simulink model "single_track"  (R2022b)
settings: Solver=VariableStepAuto  StartTime=0.0  StopTime=30  RelTol=1e-5
libraries: autolibshared x1
settings Model: Creator=ashkan  LastModifiedBy=ashkan

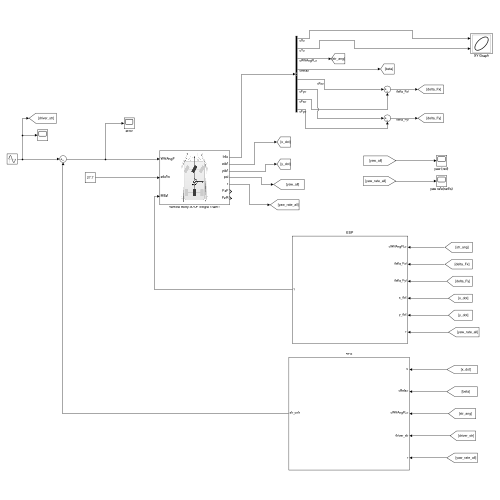
[thumbnail: Simulink's stored preview of the top-level diagram]
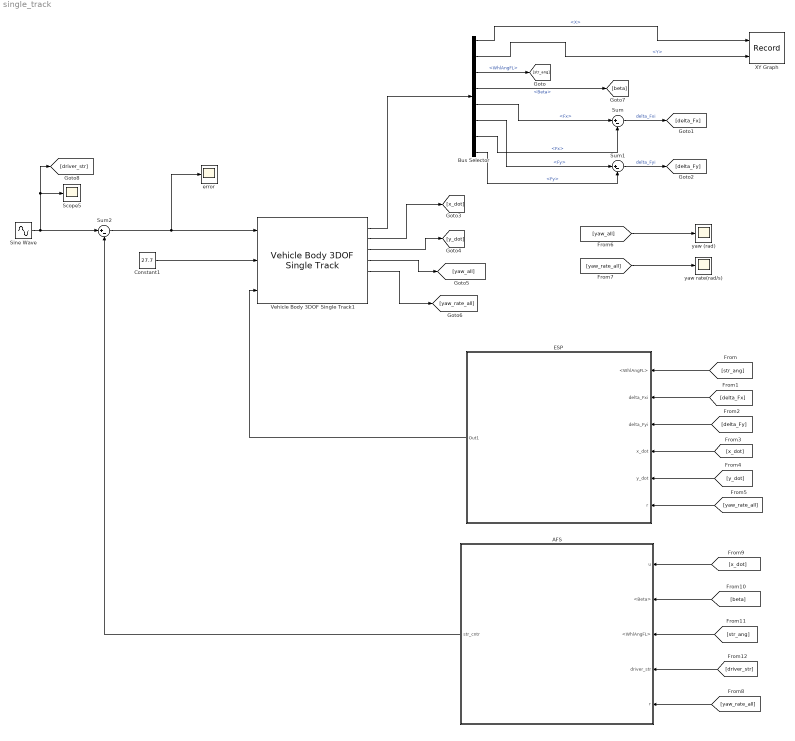
== system single_track ==
  AFS : Subsystem
  Bus Selector : BusSelector  OutputSignals=InertFrm.Cg.Disp.X,InertFrm.Cg.Disp.Y,BdyFrm.FrntAxl.Steer.WhlAngFL,BdyFrm.Cg.Ang.Beta,BdyFrm.Forces.RearAxl.Fx,BdyFrm.Forces.RearAxl.Fy,BdyFrm.Forces.FrntAxl.Fx,BdyFrm.Forces.FrntAxl.Fy
  Constant1 : Constant  Value=27.7
  ESP : Subsystem
  Scope5 : Scope
  Sine Wave : Sin  Amplitude=0.2  SampleTime=0
  Sum : Sum  Inputs=|+-
  Sum1 : Sum  Inputs=|+-
  Sum2 : Sum  Inputs=|+-
  Vehicle Body 3DOF Single Track1 : autolibshared/Vehicle Body 3DOF Single Track  trackMode=Single (bicycle)  inputMode=External longitudinal velocity  frontSteerMode=on  rearSteerMode=off  windMode=off  muMode=off  extFMode=off  extMMode=on  htchFMode=off  htchMMode=off  extXo=off  extpsio=off  extxdoto=off  extro=off  extYo=off  extTamb=off  extydoto=off  aMode=2  NF=2  NR=2  m=2000  a=1.4  b=1.6  h=0.35  dh=1  hh=0.2  X_o=0  xdot_o=0  CalphaMode=off  sigmaMode=on  d=0  hl=0  w=[1.4,1.4]  Cy_f=12e3  Cy_r=11e3  sigma_f=.1  sigma_r=.1  alpha_f_brk=[-.1 .1]  Cy_f_data=[-9e3 9e3]  alpha_r_brk=[-.1 .1]  Cy_r_data=[-9e3 9e3]  Y_o=0  ydot_o=0  Izz=4000  psi_o=0  r_o=0  Af=2  Cd=.3  Cl=.1  Cpm=.1  beta_w=[0 0.01:0.01:0.3]  Cs=[0 0.01:0.01:0.3]  Cym=[0 1e-6:0.01:0.3]  Pabs=101325  Tair=273  g=9.81  mu=1  xdot_tol=.01  Fznom=5000  Fxtire_sat=7e4  Fytire_sat=7e4  longOff=0  latOff=0  vertOff=0  wrapAng=off
  XY Graph : Record  FileSettingsInternal="{\"entries\":[{\"content\":{\"excelSettings\":{\"content\":{},\"type\":\"Streamout.ExcelSettings\"}},\"type\":\"Streamout.FileSettingStorage\",\"uuid\":\"1de5e786-87e5-4bf2-b92b-dacba8f9a9d6\"}],\"packageUris\":[\"http://schema.mathworks.com/mf0/streamout_blocks/R2020a\"],\"version\":\"1.0\"}"  Layout=[1 1]  SignalsInternal="{\"entries\":[{\"content\":{\"signals\":[{\"content\":{\"blockPath\":[\"single_track/XY Graph\"],\"channel\":[],\"dimensions\":[1],\"domain\":\"single_track/XY Graph\",\"lineColor\":\"#a2142f\",\"plots\":[1],\"port\":1,\"sid\":[],\"signalID\":17,\"signalName\":\"<X>\"},\"type\":\"RecordBlkView.Signal\",\"uuid\":\"6d30b6da-1e5d-401f-bb2f-1b54c145b824\"},{\"content\":{\"blockPath\":[\"single_track/XY Graph\"],\"channel\":[],\"dimensions\":[1],\"domain\":\"single_track/XY Graph\",\"lineColor\":\"#139fff\",\"plots\":[1],\"port\":2,\"sid\":[],\"signalID\":20,\"signalName\":\"<Y>\"},\"type\":\"RecordBlkView.Signal\",\"uuid\":\"d7a737be-39de-4a9f-801b-ad3cd6caa2f3\"}]},\"type\":\"RecordBlkView.InputSignals\",\"uuid\":\"61bda50f-d73f-43d2-879f-c24dfd1c6a79\"}],\"packageUris\":[\"http://schema.mathworks.com/mf0/streamout_blocks/R2020a\"],\"version\":\"1.0\"}"  VisualizationBindings="{\"xyplotplugin\":{\"info\":[{\"series\":[{\"bindingParametersList\":[{\"parameter\":\"X-Axis\",\"signalID\":17,\"signalName\":\"<X>\"},{\"parameter\":\"Y-Axis\",\"signalID\":20,\"signalName\":\"<Y>\"}],\"seriesID\":51129}],\"subplotID\":1}]}}"  CompatibilityTag=XY
  error : Scope
  yaw (rad) : Scope
  yaw rate(rad/s) : Scope
  wires:
  Bus Selector/7 -> Sum/2  "<Fx>"
  Bus Selector/6 -> Sum1/1  "<Fy>"
  Bus Selector/2 -> XY Graph/2  "<Y>"
  Bus Selector/5 -> Sum/1  "<Fx>"
  Bus Selector/8 -> Sum1/2  "<Fy>"
  Vehicle Body 3DOF Single Track1/5 -> [yaw_rate_all]
  Bus Selector/4 -> [beta]  "<Beta>"
  Vehicle Body 3DOF Single Track1/4 -> [yaw_all]
  Constant1/1 -> Vehicle Body 3DOF Single Track1/2
  Bus Selector/1 -> XY Graph/1  "<X>"
  Vehicle Body 3DOF Single Track1/1 -> Bus Selector/1
  Bus Selector/3 -> [str_ang]  "<WhlAngFL>"
  Sum/1 -> [delta_Fx]  "delta_Fxi"
  Sum1/1 -> [delta_Fy]  "delta_Fyi"
  Vehicle Body 3DOF Single Track1/2 -> [x_dot]
  Vehicle Body 3DOF Single Track1/3 -> [y_dot]
  ESP/1(Out1) -> Vehicle Body 3DOF Single Track1/3
  [str_ang] -> ESP/1(<WhlAngFL>)
  [delta_Fx] -> ESP/2(delta_Fxi)
  [delta_Fy] -> ESP/3(delta_Fyi)
  [x_dot] -> ESP/4(x_dot)
  [y_dot] -> ESP/5(y_dot)
  [yaw_rate_all] -> ESP/6(r)
  [yaw_rate_all] -> yaw rate(rad/s)/1
  [yaw_all] -> yaw (rad)/1
  [yaw_rate_all] -> AFS/5(r)
  [x_dot] -> AFS/1(u)
  [beta] -> AFS/2(<Beta>)
  [str_ang] -> AFS/3(<WhlAngFL>)
  [driver_str] -> AFS/4(driver_str)
  Sine Wave/1 -> Sum2/1, Scope5/1, [driver_str]
  Sum2/1 -> error/1, Vehicle Body 3DOF Single Track1/1
  AFS/1(str_cntr) -> Sum2/2

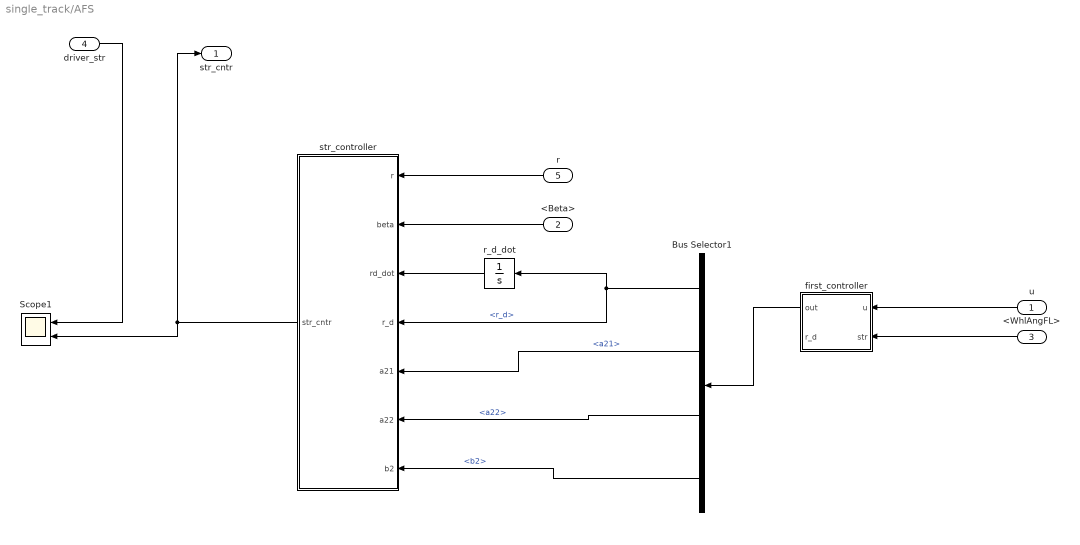
== system single_track/AFS ==
  u : Inport
  <Beta> : Inport  Port=2
  <WhlAngFL> : Inport  Port=3
  driver_str : Inport  Port=4
  r : Inport  Port=5
  Bus Selector1 : BusSelector  OutputSignals=r_d,a21,a22,b2
  Scope1 : Scope  NumInputPorts=2
  first_controller : MATLAB Function  TreatAsAtomicUnit=on
  r_d_dot : Integrator
  str_controller : MATLAB Function  TreatAsAtomicUnit=on
  str_cntr : Outport
  wires:
  driver_str/1 -> Scope1/1
  <Beta>/1 -> str_controller/2(beta)
  r/1 -> str_controller/1(r)
  first_controller/1(out) -> Bus Selector1/1
  <WhlAngFL>/1 -> first_controller/2(str)
  u/1 -> first_controller/1(u)
  Bus Selector1/2 -> str_controller/5(a21)  "<a21>"
  Bus Selector1/3 -> str_controller/6(a22)  "<a22>"
  str_controller/1(str_cntr) -> str_cntr/1, Scope1/2
  r_d_dot/1 -> str_controller/3(rd_dot)
  Bus Selector1/1 -> str_controller/4(r_d), r_d_dot/1  "<r_d>"
  Bus Selector1/4 -> str_controller/7(b2)  "<b2>"

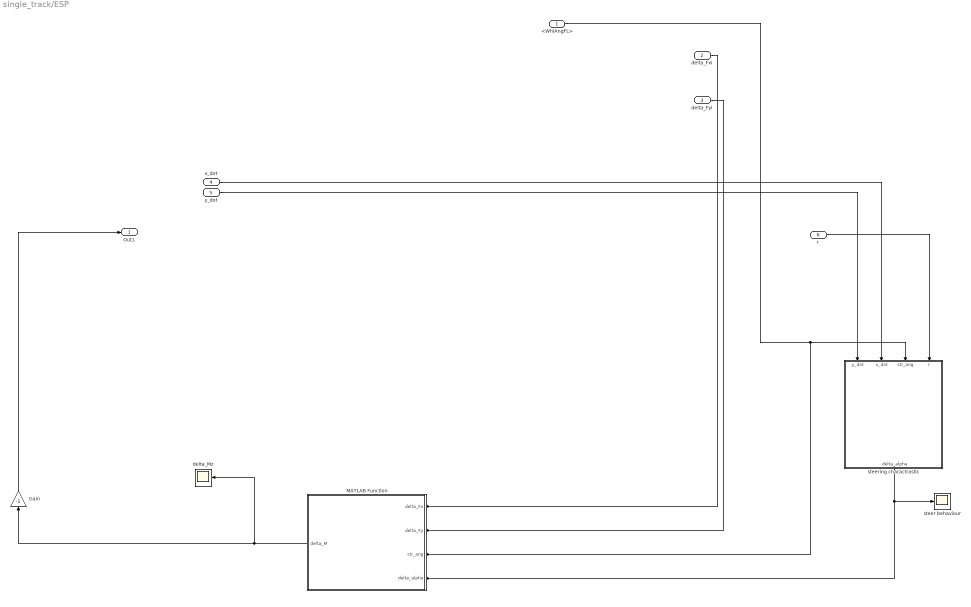
== system single_track/ESP ==
  <WhlAngFL> : Inport
  delta_Fxi : Inport  Port=2
  delta_Fyi : Inport  Port=3
  x_dot : Inport  Port=4
  y_dot : Inport  Port=5
  r : Inport  Port=6
  Gain : Gain  Gain=-1
  MATLAB Function : MATLAB Function  TreatAsAtomicUnit=on
  delta_Mz : Scope
  steer behaviour : Scope
  steering charactrastic : MATLAB Function  TreatAsAtomicUnit=on
  Out1 : Outport
  wires:
  x_dot/1 -> steering charactrastic/2(x_dot)
  delta_Fxi/1 -> MATLAB Function/1(delta_Fx)
  delta_Fyi/1 -> MATLAB Function/2(delta_Fy)
  steering charactrastic/1(delta_alpha) -> steer behaviour/1, MATLAB Function/4(delta_alpha)
  r/1 -> steering charactrastic/4(r)
  y_dot/1 -> steering charactrastic/1(y_dot)
  <WhlAngFL>/1 -> MATLAB Function/3(str_ang), steering charactrastic/3(str_ang)
  Gain/1 -> Out1/1
  MATLAB Function/1(delta_M) -> Gain/1, delta_Mz/1

== matlab function single_track/ESP/MATLAB Function ==
  data: delta_Fx input; delta_M output; delta_Fy input; str_ang input; delta_alpha input; vehicle_data parameter
function delta_M  = yaw_moment_diff(delta_Fx , delta_Fy ,  str_ang , delta_alpha , vehicle_data)

    a = vehicle_data.vehicle.Lf;
    b = vehicle_data.vehicle.Lr;
    L = vehicle_data.vehicle.L;

    if delta_alpha > 0      % over steering
        delta_Mz = (delta_Fx*(0.5*L*cos(str_ang) + a*sin(str_ang))) - (delta_Fy * (a*cos(str_ang) - 0.5*L*sin(str_ang)));


    elseif delta_alpha < 0  % under steering
        delta_Mz = (delta_Fx * 0.5*L) - (delta_Fy * b);


    else    % natural steering
        delta_Mz = 0;

    end

    delta_Mx = 0;
    delta_My = 0;

    delta_M = [delta_Mx , delta_My , delta_Mz];

end

== matlab function single_track/ESP/steering charactrastic ==
  data: y_dot input; x_dot input; delta_alpha output; str_ang input; r input; vehicle_data parameter
function delta_alpha = steer_char(y_dot , x_dot , str_ang , r , vehicle_data)

    a = vehicle_data.vehicle.Lf;
    b = vehicle_data.vehicle.Lr;

    alpha_f = atan((y_dot + a*r)/(x_dot)) - str_ang;
    alpha_r = atan((y_dot - b*r)/(x_dot));

    delta_alpha = alpha_r - alpha_f;

end

== matlab function single_track/AFS/first_controller ==
  data: out output Bus: out_rd_bus; u input; str input; vehicle_data parameter; r_d output
function [out, r_d] = r_d(u , str, vehicle_data)


% here is some simplified parameters :)
   m = vehicle_data.vehicle.m;
   a = vehicle_data.vehicle.Lf;
   b = vehicle_data.vehicle.Lr;
   izz = vehicle_data.vehicle.i_zz;
   g = vehicle_data.vehicle.g;
   L = vehicle_data.vehicle.L;
   mu = 0.2;  % --> should come from scenario
   Caf = vehicle_data.front_suspension.Ks_f ;
   Car = vehicle_data.rear_suspension.Ks_r;
   
   
% lets calculate some live parameters!!! _|_
    
   r_up_lim = 0.85 * abs(mu*g / u);
   r_ss = (2*L*Caf*Car*u)/(2*Car*Caf*L^2 - m*u^2*(a*Caf - b*Car)) * str;
   r_d = min(r_ss , r_up_lim)* sign(str);
 
   a11 = (-2*Caf - 2*Car)/(m * u);
   a12 = -1 + (2*Car*b - 2*Caf*a)/(m * u^2);
   a21 = (2*Car*b - 2*Caf*a)/izz;
   a22 = (-2*Caf*a^2 - 2*Car*b^2)/(izz * u);
   b1 = (2*Caf)/(m * u);
   b2 = (2 * Caf * a)/izz;

% outputs
   out.a11 = a11;
   out.a21 = a21;
   out.a12 = a12;
   out.a22 = a22;
   out.b1 = b1;
   out.b2 = b2;
   out.r_d = r_d;

end

== matlab function single_track/AFS/str_controller ==
  data: r input; beta input; rd_dot input; r_d input; a21 input; str_cntr output; a22 input; b2 input; AFS parameter
function str_cntr = str_controller(r, beta , rd_dot , r_d , a21 , a22 , b2, AFS)

%    lambda = AFS.lambda;
    s = r - r_d;
    lambda = AFS.lambda;
    X      = AFS.X;
    str_cntr = ((1/b2) * (-a21*beta - a22*r + rd_dot - lambda*(r - r_d))) - sign(s)*X;


end
